simulink model "UBoot_LowLevelRegler2"  (R2014a)
settings: Solver=ode45  StartTime=0.0  StopTime=inf  RelTol=1e-3
libraries: simulink x2
settings Model: Creator=Jonis  LastModifiedBy=Jonis
settings DebuggingCC: UnderspecifiedInitializationDetection=Classic

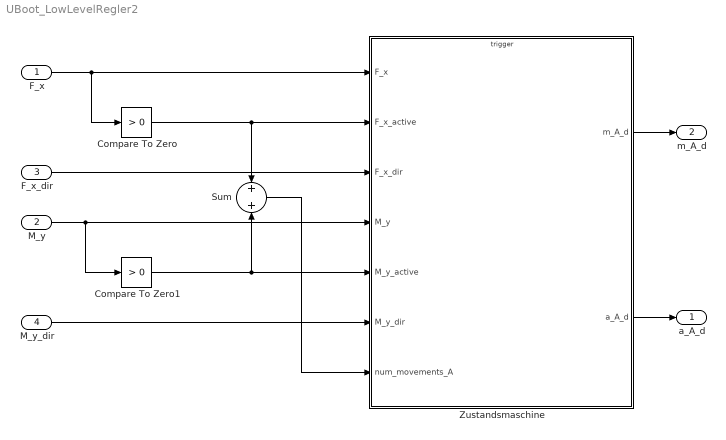
== system UBoot_LowLevelRegler2 ==
  F_x : Inport
  M_y : Inport  Port=2
  F_x_dir : Inport  Port=3
  M_y_dir : Inport  Port=4
  Compare To Zero : simulink/Logic and Bit Operations/Compare To Zero  relop=>  OutDataTypeStr=boolean
  Compare To Zero1 : simulink/Logic and Bit Operations/Compare To Zero  relop=>  OutDataTypeStr=boolean
  Sum : Sum
  Zustandsmaschine : Stateflow chart  TreatAsAtomicUnit=on
  a_A_d : Outport
  m_A_d : Outport  Port=2
  wires:
  F_x/1 -> Zustandsmaschine/1(F_x), Compare To Zero/1
  Compare To Zero/1 -> Zustandsmaschine/2(F_x_active), Sum/1
  M_y/1 -> Zustandsmaschine/4(M_y), Compare To Zero1/1
  Compare To Zero1/1 -> Sum/2, Zustandsmaschine/5(M_y_active)
  Zustandsmaschine/1(m_A_d) -> m_A_d/1
  Zustandsmaschine/2(a_A_d) -> a_A_d/1
  Sum/1 -> Zustandsmaschine/7(num_movements_A)
  F_x_dir/1 -> Zustandsmaschine/3(F_x_dir)
  M_y_dir/1 -> Zustandsmaschine/6(M_y_dir)

== stateflow chart UBoot_LowLevelRegler2/Zustandsmaschine ==
  data: A_angle_negative_force constant double; A_angle_negative_torque constant double; A_angle_positive_force constant double; A_angle_positive_torque constant double; F_x input; F_x_active input; F_x_dir input; M_y input; M_y_active input; M_y_dir input; num_movements_A input; switch_time constant double; m_A_d output double; a_A_d output double
  events: s input RISING_EDGE_EVENT
